simulink model "hw7"  (R2024a)
settings: Solver=VariableStepAuto  StartTime=0.0  StopTime=10.0  RelTol=1e-3
settings RTWCC: GPUComputeCapability=3.5

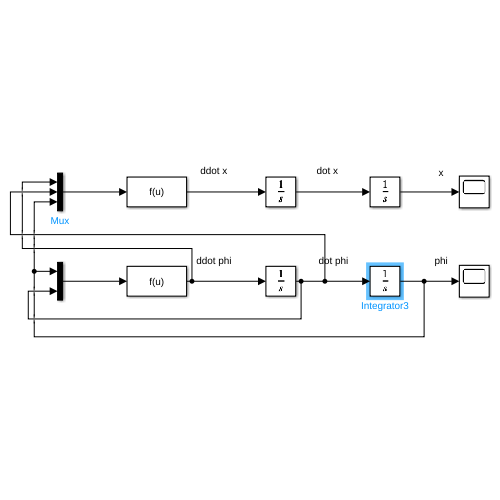
[thumbnail: Simulink's stored preview of the top-level diagram]
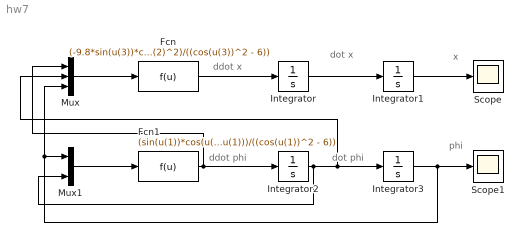
== system hw7 ==
  note: ddot x
  note: ddot phi
  note: dot phi
  note: phi
  note: x
  note: dot x
  Fcn : Fcn  Expr=(-9.8*sin(u(3))*cos(u(3))- sin(u(3))*u(2)^2)/((cos(u(3))^2 - 6))
  Fcn1 : Fcn  Expr=(sin(u(1))*cos(u(1))*(u(2))^2+58.8* sin(u(1)))/((cos(u(1))^2 - 6))
  Integrator : Integrator
  Integrator1 : Integrator  InitialCondition=0.5
  Integrator2 : Integrator
  Integrator3 : Integrator  InitialCondition=45*pi/180
  Mux : Mux  Inputs=3
  Mux1 : Mux  Inputs=2
  Scope : Scope
  Scope1 : Scope
  wires:
  Integrator/1 -> Integrator1/1
  Integrator2/1 -> Mux1/2, Mux/2, Integrator3/1
  Fcn/1 -> Integrator/1
  Fcn1/1 -> Mux/1, Integrator2/1
  Integrator3/1 -> Scope1/1, Mux1/1, Mux/3
  Mux/1 -> Fcn/1
  Mux1/1 -> Fcn1/1
  Integrator1/1 -> Scope/1
